simulink model "TRN_V3_2_CodeGen"  (R2022a)
settings: Solver=FixedStepAuto  StartTime=0.0  StopTime=300  FixedStep=0.04  RelTol=1e-3
PreLoadFcn:
  | load('BusStructureTRNsensor.mat');
  | addpath('C:/MAP');
InitFcn:
  | %load TRNDataBusPILS.mat
  | %addpath(genpath(cd))
  | 
  | %load('TPF_WHOLESIM_INPUT_SCENARIOS_AGCAS_N35_10E127_70.mat');
  | 
  | % Add DataBus Path
  | addpath(',,/');
  | addpath('../MAP/');
  | addpath('../MAP/MAP_DB');
  | addpath('../MAP/DVOF');
  | addpath(genpath(cd));
  | load('BusStructureTRN.mat');
undefined symbols (not defined in the file or in its folder): Altitude_INS, Latitude_INS, Longitude_INS, TRN, TRNlib
libraries: simulink_extras x23, aerolibconvert2 x6, sharedtransform x4, dspstat3 x2
(part 2 of 3)

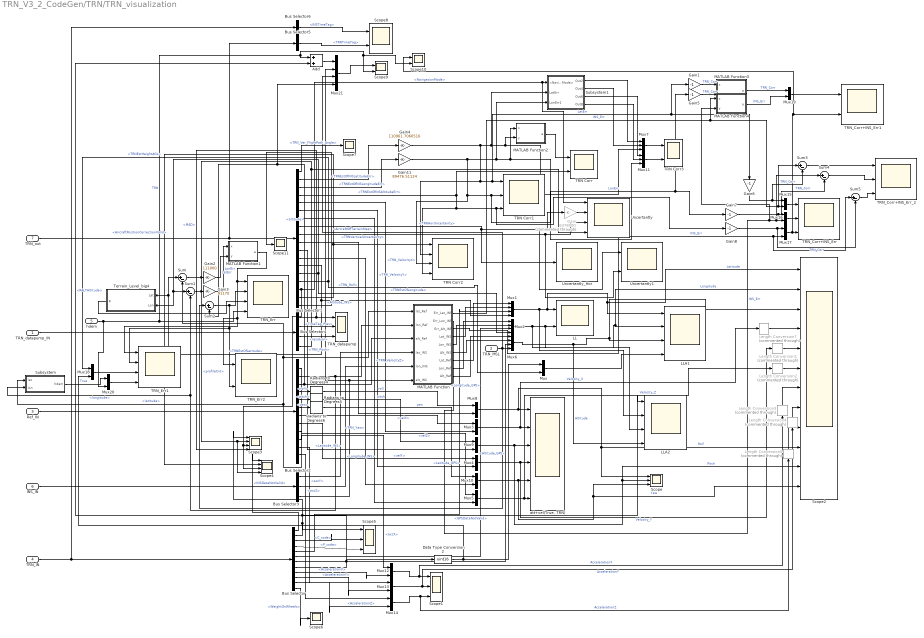
== system TRN_V3_2_CodeGen/TRN/TRN_visualization  ==
  TRN_datapump_IN : Inport
  TRN_MSL : Inport  Port=2
  Ref_IN : Inport  Port=3
  TRN_IN : Inport  Port=4
  hdem : Inport  Port=5
  INS_IN : Inport  Port=6
  TRN_out : Inport  Port=7
  Add : Sum
  Bus Selector : BusSelector  OutputSignals=INSDataNotValid,GPSDataNotValid,C_code,P_code,Latitude_GPS,Longitude_GPS,Altitude_GPS,RALTAltitude,AccelerationX,AccelerationY,AccelerationZ,WeightOnWheels
  Bus Selector1 : BusSelector  OutputSignals=TRN_Ver_FlightPath_Angle,TRNEstOfINSLatitudeErr,TRNEstOfINSLongitudeErr,TRNEstOfINSAltitudeErr,TRN_VelocityX,TRN_VelocityY,TRN_VelocityZ,TRNHorUncertainty,TRNVerticalUncertainty,TRN_Roll,TRN_Pitch,TRN_Yaw,TRNEstOfLatitude,TRNEstOfLongitude,TRNEstHeightAGL,NavigationMode,AircraftPositionCorrectionValid,AircraftOffTerrainMap
  Bus Selector2 : BusSelector  OutputSignals=latitude,longitude,altitude,roll,pitch,yaw,velX,velY,velZ,accX,accY,accZ
  Bus Selector3 : BusSelector  OutputSignals=Latitude_INS,Longitude_INS,Altitude_INS
  Bus Selector4 : BusSelector  OutputSignals=MAD,TimeTag_Prev,residual,profileCnt
  Bus Selector5 : BusSelector  OutputSignals=TRNTimeTag
  Bus Selector6 : BusSelector  OutputSignals=INSTimeTag
  Data Type Conversion2 : DataTypeConversion  OutDataTypeStr=uint16  SaturateOnIntegerOverflow=off  RndMeth=Floor
  Gain : Gain  Commented=through  Gain=6378000
  Gain{1,5..8} (5 alike) : Gain  Gain=-1
  Gain11 : Gain  Gain=89476.51124
  Gain2 : Gain  Gain=111000
  Gain3 : Gain  Gain=91170
  Gain4 : Gain  Gain=110961.7060516
  LL : Scope  NumInputPorts=2
  LLA1 : Scope  NumInputPorts=4
  LLA2 : Scope  NumInputPorts=4
  Length Conversion{1..5,7} (6 alike) : aerolibconvert2/Length Conversion  Commented=through  IU=m  OU=ft
  MATLAB Function : MATLAB Function  TreatAsAtomicUnit=on
  MATLAB Function1 : MATLAB Function  TreatAsAtomicUnit=on
  MATLAB Function2 : MATLAB Function  TreatAsAtomicUnit=on
  MATLAB Function3 : MATLAB Function  TreatAsAtomicUnit=on
  MATLAB Function4 : MATLAB Function  TreatAsAtomicUnit=on
  Mux{,3..5,8..10,12..20} (16 alike) : Mux  Inputs=2
  Mux{1..2,6,21} (4 alike) : Mux
  Mux11 : Mux  Inputs=3
  Mux7 : Mux  Inputs=3
  Radians to Degrees4 : simulink_extras/Transformations/Radians to Degrees
  Radians to Degrees5 : simulink_extras/Transformations/Radians to Degrees
  Radians to Degrees6 : simulink_extras/Transformations/Radians to Degrees
  Scope : Scope  NumInputPorts=3
  Scope1 : Scope  NumInputPorts=3
  Scope10 : Scope  NumInputPorts=2
  Scope11 : Scope
  Scope2 : Scope  NumInputPorts=12
  Scope3 : Scope  NumInputPorts=4
  Scope4 : Scope  NumInputPorts=4
  Scope5 : Scope  NumInputPorts=3
  Scope6 : Scope
  Scope7 : Scope
  Scope8 : Scope  NumInputPorts=2
  Scope9 : Scope  NumInputPorts=2
  Subsystem : Subsystem
  Subsystem1 : Subsystem
  Sum{,1..5} (6 alike) : Sum  Inputs=|+-
  TRN Corr : Scope  NumInputPorts=2
  TRN Corr1 : Scope  NumInputPorts=3
  TRN Corr2 : Scope  NumInputPorts=4
  TRN Corr3 : Scope  NumInputPorts=2
  TRN_Corr+INS_Err : Scope  NumInputPorts=3
  TRN_Corr+INS_Err1 : Scope  NumInputPorts=2
  TRN_Corr+INS_Err_2 : Scope  NumInputPorts=3
  TRN_Err : Scope  NumInputPorts=4
  TRN_Err1 : Scope  NumInputPorts=4
  TRN_Err2 : Scope  NumInputPorts=2
  TRN_datapump : Scope  NumInputPorts=3
  Terrain_Level_big4 : MATLAB Function  TreatAsAtomicUnit=on
  Uncertantly : Scope  NumInputPorts=4
  Uncertantly1 : Scope  NumInputPorts=2
  Uncertantly_Hor : Scope
  "att+vel(True, TRN)" : Scope  NumInputPorts=6
  wires:
  Sum3/1 -> TRN_Corr+INS_Err_2/1
  Sum4/1 -> TRN_Corr+INS_Err_2/2
  Sum5/1 -> TRN_Corr+INS_Err_2/3
  Gain8/1 -> Mux17/1, Sum5/2  "TRN_Corr"
  Gain7/1 -> Mux16/1, Sum4/2  "TRN_Corr"
  Gain6/1 -> Mux15/1, Sum3/2  "TRN_Corr"
  MATLAB Function/3(Err_Alt_INS) -> Mux17/2, Sum5/1  "INS_Err"
  Mux17/1 -> Scope10/1, TRN_Corr+INS_Err1/2, TRN_Corr+INS_Err/3
  MATLAB Function/2(Err_Lon_INS) -> Mux16/2, Sum4/1, MATLAB Function4/2(y)  "INS_Err"
  Mux16/1 -> TRN_Corr+INS_Err/2
  Mux15/1 -> TRN_Corr+INS_Err/1
  MATLAB Function/1(Err_Lat_INS) -> Mux15/2, Sum3/1, MATLAB Function4/1(x)  "INS_Err"
  Bus Selector/4 -> Scope5/3  "<P_code>"
  Bus Selector/3 -> Scope5/2  "<C_code>"
  Bus Selector/7 -> Mux6/3  "<Altitude_GPS>"
  Bus Selector/6 -> Mux2/3  "<Longitude_GPS>"
  Bus Selector/5 -> Mux1/3  "<Latitude_GPS>"
  Length Conversion5/1 -> Scope2/9
  Length Conversion4/1 -> Scope2/8
  Length Conversion3/1 -> Scope2/7
  Length Conversion2/1 -> Scope2/6
  Length Conversion1/1 -> Scope2/5
  Length Conversion7/1 -> Scope2/4
  Bus Selector/1 -> Scope4/1  "<INSDataNotValid>"
  Bus Selector4/4 -> Uncertantly/4, Scope3/2, Scope4/4  "<profileCnt>"
  MATLAB Function1/1(a) -> TRN_Err2/1, TRN_Err1/1, TRN_Err/1
  Bus Selector/2 -> Scope3/1, LLA2/1, Scope5/1  "<GPSDataNotValid>"
  hdem/1 -> Mux20/2, Scope10/2, Scope9/2, Add/1, TRN_Err/4  "TRN"
  Terrain_Level_big4/1(R) -> TRN_Err/3
  Bus Selector1/17 -> TRN Corr2/1, Scope4/2  "<AircraftPositionCorrectionValid>"
  Bus Selector1/5 -> Mux3/2  "<TRN_VelocityX>"
  Mux14/1 -> Scope1/3, Length Conversion5/1  "AccelerationZ"
  Bus Selector/11 -> Mux14/2  "<AccelerationZ>"
  Bus Selector2/12 -> Mux14/1  "<accZ>"
  Bus Selector2/11 -> Mux13/1  "<accY>"
  Bus Selector/10 -> Mux13/2  "<AccelerationY>"
  Mux13/1 -> Scope1/2, Length Conversion4/1  "AccelerationY"
  Bus Selector/9 -> Mux12/2  "<AccelerationX>"
  Bus Selector2/10 -> Mux12/1  "<accX>"
  Mux12/1 -> Scope1/1, Length Conversion3/1  "AccelerationX"
  Mux6/1 -> LLA1/3, Scope2/3, LLA2/4  "Altitude"
  Mux/1 -> LLA1/4
  TRN_IN/1 -> Bus Selector/1, Bus Selector6/1
  Ref_IN/1 -> Bus Selector2/1
  TRN_out/1 -> Bus Selector5/1, Bus Selector1/1
  Gain3/1 -> MATLAB Function1/1(x)  "LonErr"
  Subsystem1/1(Out2) -> Mux7/1
  Mux11/1 -> TRN Corr3/2
  Bus Selector1/9 -> Uncertantly/3, Uncertantly1/2  "<TRNVerticalUncertainty>"
  Bus Selector1/14 -> Mux2/4, Sum1/1, Terrain_Level_big4/2(Lon)  "<TRNEstOfLongitude>"
  Radians to Degrees5/1 -> Mux9/1  "pitch"
  Radians to Degrees4/1 -> Mux8/1  "roll"
  Bus Selector2/7 -> Mux3/1  "<velX>"
  MATLAB Function/6(Alt_INS) -> Mux6/2
  Bus Selector1/12 -> Mux10/2  "<TRN_Yaw>"
  Bus Selector1/11 -> Mux9/2  "<TRN_Pitch>"
  Mux3/1 -> "att+vel(True, TRN)"/2, Length Conversion7/1  "Velocity_X"
  Bus Selector1/10 -> Mux8/2  "<TRN_Roll>"
  Bus Selector3/3 -> Mux21/2, MATLAB Function/6(alt_INS)  "<Altitude_INS>"
  Bus Selector2/9 -> Mux5/1  "<velZ>"
  Mux4/1 -> "att+vel(True, TRN)"/4, Length Conversion1/1  "Velocity_Y"
  Mux1/1 -> LL/1, LLA1/1, Scope2/1, LLA2/2  "Latitude"
  Mux5/1 -> "att+vel(True, TRN)"/6, Length Conversion2/1  "Velocity_Z"
  Bus Selector2/3 -> MATLAB Function/3(alt_Ref), Mux21/4, Sum2/2  "<altitude>"
  Bus Selector1/4 -> TRN Corr2/4, TRN Corr1/3, Gain8/1, TRN Corr/2  "<TRNEstOfINSAltitudeErr>"
  TRN_datapump_IN/1 -> Bus Selector4/1
  Mux2/1 -> LL/2, LLA1/2, Scope2/2, LLA2/3  "Longitude"
  MATLAB Function/9(Alt_Ref) -> Mux6/1
  Gain11/1 -> Mux11/3, MATLAB Function2/1(x), Subsystem1/3(LonErr1), TRN Corr1/2, Gain7/1, Gain5/1, TRN Corr2/3  "LonErr"
  MATLAB Function/4(Lat_INS) -> Mux1/2
  Bus Selector3/2 -> MATLAB Function/5(lon_INS)  "<Longitude_INS>"
  Radians to Degrees6/1 -> Mux10/1  "yaw"
  Bus Selector4/2 -> TRN_datapump/2  "<TimeTag_Prev>"
  MATLAB Function/8(Lon_Ref) -> Mux2/1
  Bus Selector2/6 -> Radians to Degrees6/1  "<yaw>"
  MATLAB Function2/1(a) -> TRN Corr/1
  Bus Selector/8 -> Add/2, Data Type Conversion2/1  "<RALTAltitude>"
  Bus Selector1/16 -> Scope3/3, Scope4/3, Uncertantly/1, Subsystem1/1(<NavigationMode>)  "<NavigationMode>"
  Sum2/1 -> TRN_Err1/2, TRN_Err2/2, TRN_Err/2
  Bus Selector2/5 -> Radians to Degrees5/1  "<pitch>"
  Mux7/1 -> TRN Corr3/1
  INS_IN/1 -> Bus Selector3/1
  Bus Selector4/1 -> TRN_datapump/1, Scope3/4  "<MAD>"
  Bus Selector1/3 -> Gain11/1  "<TRNEstOfINSLongitudeErr>"
  Bus Selector1/6 -> Mux4/2  "<TRN_VelocityY>"
  Bus Selector3/1 -> MATLAB Function/4(lat_INS)  "<Latitude_INS>"
  Subsystem1/3(Out6) -> Mux11/1
  Mux8/1 -> "att+vel(True, TRN)"/1, Scope/1, Scope2/10  "Roll"
  TRN_MSL/1 -> Mux21/3, Sum2/1, Mux6/4
  Bus Selector1/15 -> Mux/2, Mux18/1  "<TRNEstHeightAGL>"
  MATLAB Function/7(Lat_Ref) -> Mux1/1
  Mux9/1 -> "att+vel(True, TRN)"/3, Scope/2, Scope2/11  "Pitch"
  Subsystem1/2(Out4) -> Mux7/2
  Sum1/1 -> Gain3/1
  Bus Selector1/7 -> Mux5/2  "<TRN_VelocityZ>"
  Bus Selector1/2 -> Gain4/1  "<TRNEstOfINSLatitudeErr>"
  Bus Selector2/2 -> Subsystem/2(lon), Sum1/2, MATLAB Function/2(lon_Ref)  "<longitude>"
  Subsystem1/4(Out8) -> Mux11/2
  Gain2/1 -> MATLAB Function1/2(y)  "LatErr"
  Gain4/1 -> Mux7/3, MATLAB Function2/2(y), Subsystem1/2(LatErr), TRN Corr1/1, Gain6/1, Gain1/1, TRN Corr2/2  "LatErr"
  Bus Selector2/8 -> Mux4/1  "<velY>"
  MATLAB Function/5(Lon_INS) -> Mux2/2
  Bus Selector4/3 -> TRN_datapump/3  "<residual>"
  Bus Selector1/8 -> Uncertantly_Hor/1, Gain/1, Uncertantly1/1  "<TRNHorUncertainty>"
  Sum/1 -> Gain2/1
  Mux10/1 -> "att+vel(True, TRN)"/5, Scope2/12, Scope/3  "Yaw"
  Bus Selector2/1 -> MATLAB Function/1(lat_Ref), Sum/2, Subsystem/1(lat)  "<latitude>"
  Bus Selector2/4 -> Radians to Degrees4/1  "<roll>"
  Bus Selector1/13 -> Sum/1, Terrain_Level_big4/1(Lat), Mux1/4  "<TRNEstOfLatitude>"
  Bus Selector/12 -> Scope6/1  "<WeightOnWheels>"
  Bus Selector1/1 -> Scope7/1  "<TRN_Ver_FlightPath_Angle>"
  Mux18/1 -> TRN_Err1/3
  Data Type Conversion2/1 -> Mux/1, Mux18/2
  Mux19/1 -> TRN_Corr+INS_Err1/1
  MATLAB Function4/1(a) -> Mux19/2  "INS_Err"
  MATLAB Function3/1(a) -> Mux19/1  "TRN_Corr"
  Gain1/1 -> MATLAB Function3/1(x)  "TRN_Corr"
  Gain5/1 -> MATLAB Function3/2(y)  "TRN_Corr"
  Mux20/1 -> TRN_Err1/4
  Subsystem/1(hdem) -> Mux20/1  "True"
  Bus Selector6/1 -> Scope8/1  "<INSTimeTag>"
  Bus Selector5/1 -> Scope8/2  "<TRNTimeTag>"
  Add/1 -> Mux21/1
  Mux21/1 -> Scope9/1
  Gain/1 -> Uncertantly/2
  Bus Selector1/18 -> Scope11/1  "<AircraftOffTerrainMap>"

== system TRN_V3_2_CodeGen/TRN/Terrain_Func ==
  lat : Inport
  lon : Inport  Port=2
  CheckOffTerrainMap : MATLAB Function  TreatAsAtomicUnit=on
  MATLAB Function : MATLAB Function  Commented=on  TreatAsAtomicUnit=on
  Terminator : Terminator
  Terrain_roughness : MATLAB Function  TreatAsAtomicUnit=on
  UpdateCache : MATLAB Function  TreatAsAtomicUnit=on
  updateFlag : MATLAB Function  TreatAsAtomicUnit=on
  hdem : Outport
  Updateflag : Outport  Port=2
  AircraftOffTerrainMap : Outport  Port=3
  wires:
  lat/1 -> UpdateCache/1(lat), Terrain_roughness/1(Lat)
  UpdateCache/2(hDEM) -> CheckOffTerrainMap/1(hDEM), hdem/1
  lon/1 -> UpdateCache/2(lon), Terrain_roughness/2(Lon)
  Terrain_roughness/1(R) -> updateFlag/2(roughness)
  updateFlag/1(UpdateFlag) -> Updateflag/1
  CheckOffTerrainMap/1(AircraftOffTerrainMap) -> updateFlag/1(AircraftOffTerrainMap), AircraftOffTerrainMap/1
  UpdateCache/1(result) -> Terminator/1

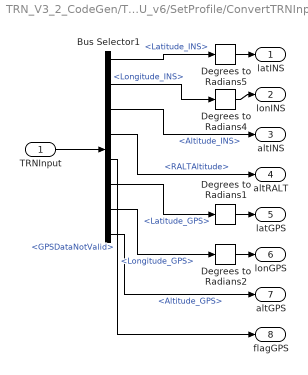
== system TRN_V3_2_CodeGen/TRN/ModeManagementCSU_v6/SetProfile/ConvertTRNInput ==
  TRNInput : Inport  OutDataTypeStr=Bus: TRNInput
  Bus Selector1 : BusSelector  OutputSignals=Latitude_INS,Longitude_INS,Altitude_INS,RALTAltitude,GPSDataNotValid,Latitude_GPS,Longitude_GPS,Altitude_GPS
  Degrees to Radians{1..2,4..5} (4 alike) : simulink_extras/Transformations/Degrees to Radians
  latINS : Outport  VectorParamsAs1DForOutWhenUnconnected=off
  lonINS : Outport  Port=2  VectorParamsAs1DForOutWhenUnconnected=off
  altINS : Outport  Port=3  VectorParamsAs1DForOutWhenUnconnected=off
  altRALT : Outport  Port=4  VectorParamsAs1DForOutWhenUnconnected=off
  latGPS : Outport  Port=5  VectorParamsAs1DForOutWhenUnconnected=off
  lonGPS : Outport  Port=6  VectorParamsAs1DForOutWhenUnconnected=off
  altGPS : Outport  Port=7  VectorParamsAs1DForOutWhenUnconnected=off
  flagGPS : Outport  Port=8  VectorParamsAs1DForOutWhenUnconnected=off
  wires:
  Bus Selector1/2 -> Degrees to Radians4/1  "<Longitude_INS>"
  Bus Selector1/1 -> Degrees to Radians5/1  "<Latitude_INS>"
  Bus Selector1/4 -> altRALT/1  "<RALTAltitude>"
  Degrees to Radians4/1 -> lonINS/1
  Degrees to Radians5/1 -> latINS/1
  TRNInput/1 -> Bus Selector1/1
  Bus Selector1/3 -> altINS/1  "<Altitude_INS>"
  Bus Selector1/5 -> flagGPS/1  "<GPSDataNotValid>"
  Bus Selector1/6 -> Degrees to Radians1/1  "<Latitude_GPS>"
  Bus Selector1/7 -> Degrees to Radians2/1  "<Longitude_GPS>"
  Bus Selector1/8 -> altGPS/1  "<Altitude_GPS>"
  Degrees to Radians2/1 -> lonGPS/1
  Degrees to Radians1/1 -> latGPS/1

== system TRN_V3_2_CodeGen/TRN/ModeManagementCSU_v6/TrackingCSUMeasurement/residualValidCheck2 ==
  TRNDatapump : Inport
  Bus Selector7 : BusSelector  OutputSignals=residual
  Data Type Conversion2 : DataTypeConversion  OutDataTypeStr=boolean  SaturateOnIntegerOverflow=off  RndMeth=Floor
  Gain2 : Gain  Gain=3
  StdDev : MATLAB Function  TreatAsAtomicUnit=on
  Unit Delay3 : UnitDelay  SampleTime=-1  HasFrameUpgradeWarning=on
  residualCheck : MATLAB Function  TreatAsAtomicUnit=on
  residualValid : Outport
  wires:
  Data Type Conversion2/1 -> residualValid/1
  residualCheck/1(residualValid) -> Data Type Conversion2/1
  StdDev/1(std) -> Gain2/1
  Gain2/1 -> residualCheck/2(sigma_3)
  residualCheck/2(count) -> Unit Delay3/1
  TRNDatapump/1 -> Bus Selector7/1
  Unit Delay3/1 -> residualCheck/3("count ")
  Bus Selector7/1 -> StdDev/1(x), residualCheck/1(residual)  "<residual>"

== system TRN_V3_2_CodeGen/TRN/TRN_visualization /Subsystem ==
  lat : Inport
  lon : Inport  Port=2
  MATLAB Function : MATLAB Function  Commented=on  TreatAsAtomicUnit=on
  UpdateCache : MATLAB Function  TreatAsAtomicUnit=on
  hdem : Outport
  wires:
  lat/1 -> UpdateCache/1(lat)
  UpdateCache/2(hDEM) -> hdem/1
  lon/1 -> UpdateCache/2(lon)

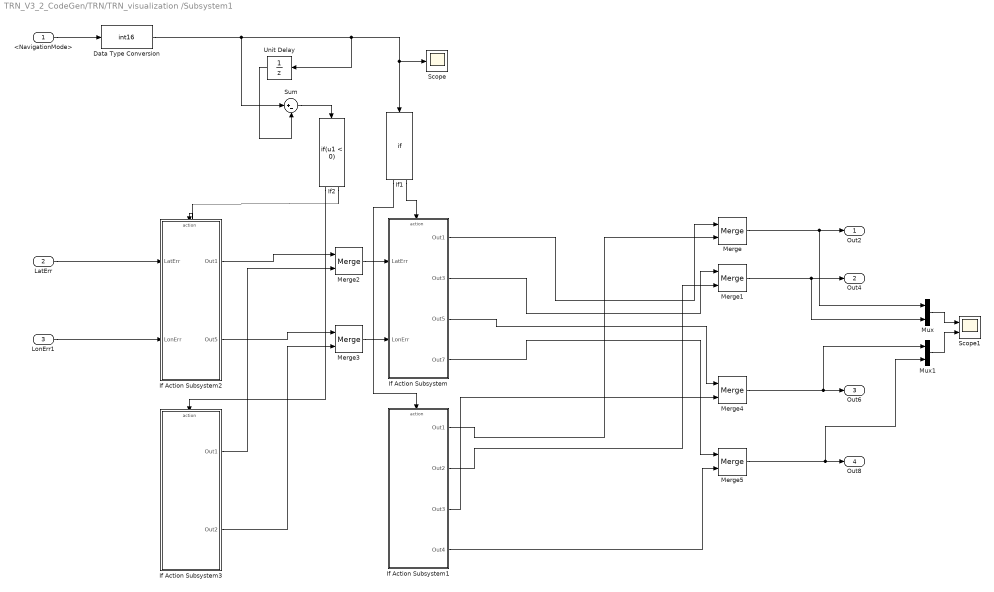
== system TRN_V3_2_CodeGen/TRN/TRN_visualization /Subsystem1 ==
  <NavigationMode> : Inport
  LatErr : Inport  Port=2
  LonErr1 : Inport  Port=3
  Data Type Conversion : DataTypeConversion  OutDataTypeStr=int16  SaturateOnIntegerOverflow=off  RndMeth=Floor
  If Action Subsystem : Subsystem  TreatAsAtomicUnit=on
  If Action Subsystem1 : Subsystem  TreatAsAtomicUnit=on
  If Action Subsystem2 : Subsystem  TreatAsAtomicUnit=on
  If Action Subsystem3 : Subsystem  TreatAsAtomicUnit=on
  If1 : If
  If2 : If  IfExpression=u1 < 0
  Merge{,1..5} (6 alike) : Merge
  Mux : Mux  Inputs=2
  Mux1 : Mux  Inputs=2
  Scope : Scope
  Scope1 : Scope  NumInputPorts=2
  Sum : Sum  Inputs=|+-
  Unit Delay : UnitDelay  SampleTime=-1  HasFrameUpgradeWarning=on
  Out2 : Outport
  Out4 : Outport  Port=2
  Out6 : Outport  Port=3
  Out8 : Outport  Port=4
  wires:
  If Action Subsystem3/2(Out2) -> Merge3/2
  If Action Subsystem2/2(Out5) -> Merge3/1
  If Action Subsystem3/1(Out1) -> Merge2/2
  If Action Subsystem2/1(Out1) -> Merge2/1
  Merge3/1 -> If Action Subsystem/2(LonErr)
  Merge2/1 -> If Action Subsystem/1(LatErr)
  LonErr1/1 -> If Action Subsystem2/2(LonErr)
  LatErr/1 -> If Action Subsystem2/1(LatErr)
  If2/1 -> If Action Subsystem3/Action
  If2/2 -> If Action Subsystem2/Action
  Sum/1 -> If2/1
  Unit Delay/1 -> Sum/2
  Mux1/1 -> Scope1/2
  Mux/1 -> Scope1/1
  <NavigationMode>/1 -> Data Type Conversion/1
  If Action Subsystem1/4(Out4) -> Merge5/2
  If Action Subsystem1/3(Out3) -> Merge4/2
  If Action Subsystem/4(Out7) -> Merge5/1
  If Action Subsystem/3(Out5) -> Merge4/1
  If Action Subsystem/2(Out3) -> Merge1/1
  Merge1/1 -> Out4/1, Mux/2
  Merge/1 -> Out2/1, Mux/1
  If1/1 -> If Action Subsystem1/Action
  If Action Subsystem1/1(Out1) -> Merge/2
  If Action Subsystem1/2(Out2) -> Merge1/2
  Data Type Conversion/1 -> Sum/1, Scope/1, If1/1, Unit Delay/1
  Merge4/1 -> Out6/1, Mux1/1
  Merge5/1 -> Out8/1, Mux1/2
  If1/2 -> If Action Subsystem/Action
  If Action Subsystem/1(Out1) -> Merge/1

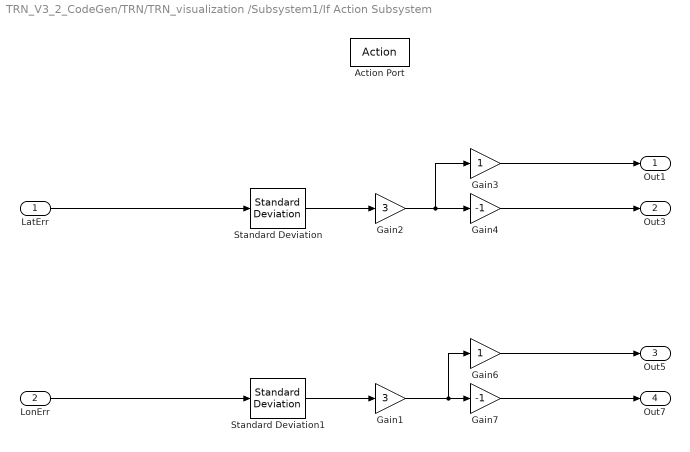
== system TRN_V3_2_CodeGen/TRN/TRN_visualization /Subsystem1/If Action Subsystem ==
  LatErr : Inport
  LonErr : Inport  Port=2
  Action Port : ActionPort
  Gain1 : Gain  Gain=3
  Gain2 : Gain  Gain=3
  Gain3 : Gain
  Gain4 : Gain  Gain=-1
  Gain6 : Gain
  Gain7 : Gain  Gain=-1
  Standard Deviation : dspstat3/Standard Deviation  run=on  directionMode=Entire input  dimension=1  reset_popup=None  roiEnable=off  roiType=Rectangles  roiPortion=Entire ROI  roiOutput=Individual statistics for each ROI  roiFlag=off
      settings: SourceProductBaseCode=DS
  Standard Deviation1 : dspstat3/Standard Deviation  run=on  directionMode=Entire input  dimension=1  reset_popup=None  roiEnable=off  roiType=Rectangles  roiPortion=Entire ROI  roiOutput=Individual statistics for each ROI  roiFlag=off
      settings: SourceProductBaseCode=DS
  Out1 : Outport
  Out3 : Outport  Port=2
  Out5 : Outport  Port=3
  Out7 : Outport  Port=4
  wires:
  LatErr/1 -> Standard Deviation/1
  LonErr/1 -> Standard Deviation1/1
  Gain6/1 -> Out5/1
  Gain2/1 -> Gain4/1, Gain3/1
  Gain7/1 -> Out7/1
  Standard Deviation1/1 -> Gain1/1
  Standard Deviation/1 -> Gain2/1
  Gain3/1 -> Out1/1
  Gain4/1 -> Out3/1
  Gain1/1 -> Gain7/1, Gain6/1

== system TRN_V3_2_CodeGen/TRN/TRN_visualization /Subsystem1/If Action Subsystem1 ==
  Action Port : ActionPort
  Constant : Constant  Value=0
  Out1 : Outport
  Out2 : Outport  Port=2
  Out3 : Outport  Port=3
  Out4 : Outport  Port=4
  wires:
  Constant/1 -> Out4/1, Out3/1, Out2/1, Out1/1

== system TRN_V3_2_CodeGen/TRN/TRN_visualization /Subsystem1/If Action Subsystem2 ==
  LatErr : Inport
  LonErr : Inport  Port=2
  Action Port : ActionPort
  Out1 : Outport
  Out5 : Outport  Port=2
  wires:
  LonErr/1 -> Out5/1
  LatErr/1 -> Out1/1

== system TRN_V3_2_CodeGen/TRN/TRN_visualization /Subsystem1/If Action Subsystem3 ==
  Action Port : ActionPort
  Constant : Constant  Value=0
  Out1 : Outport
  Out2 : Outport  Port=2
  wires:
  Constant/1 -> Out2/1, Out1/1

== matlab function TRN_V3_2_CodeGen/TRN/Terrain_Func/CheckOffTerrainMap ==
  data: hDEM input; AircraftOffTerrainMap output
function AircraftOffTerrainMap = CheckOffTerrainMap(hDEM)

if(hDEM == -1)
    AircraftOffTerrainMap = true;
else
    AircraftOffTerrainMap = false;
end

end

== matlab function TRN_V3_2_CodeGen/TRN/ModeManagementCSU_v6/StoreProfile/SetProfile function ==
  data: batchProfile input; batchProfile output; profileCnt input; profileCnt output; gridSize input; flagINS input
function [batchProfile, profileCnt] = SetProfile(batchProfile, profileCnt, gridSize, flagINS)

if(profileCnt >= 20)
      
    profileCnt = uint32(19);
    
    for i = 0:profileCnt-1
   
        for j = 1 : (3 + (gridSize + gridSize + 1) * (gridSize + gridSize + 1))
            batchProfile(i * (3 + (gridSize + gridSize + 1) * (gridSize + gridSize + 1)) + j) = batchProfile((i+1) * (3 + (gridSize + gridSize + 1) * (gridSize + gridSize + 1)) + j);
        end
    end
            
end

if flagINS == 0
    profileCnt = profileCnt + 1;
else
    profileCnt = uint32(0);
end


end

== matlab function TRN_V3_2_CodeGen/TRN/TRNCorrCheck ==
  data: latINS input; TRNEstOfLatErr output; lonINS input; altINS input; TRNEstOfLonErr output; TRNEstOfaltErr output; roll input; pitch input; GPSDataNotvalid input; NotCorrFlag input; NotCorrFlag output
function [TRNEstOfLatErr, TRNEstOfLonErr, TRNEstOfaltErr,NotCorrFlag] = TRNCorrCheck(latINS, lonINS, altINS, roll, pitch, GPSDataNotvalid, NotCorrFlag)

if GPSDataNotvalid == true
    if abs(roll) > 15 || abs(pitch) > 15
        TRNEstOfLatErr_temp = latINS;
        TRNEstOfLonErr_temp = lonINS;
        TRNEstOfaltErr_temp = altINS;
        TRNEstOfLatErr = TRNEstOfLatErr_temp;
        TRNEstOfLonErr = TRNEstOfLonErr_temp;
        TRNEstOfaltErr = TRNEstOfaltErr_temp;
        NotCorrFlag = 1;
    else
        TRNEstOfLatErr = latINS;
        TRNEstOfLonErr = lonINS;
        TRNEstOfaltErr = altINS;
        TRNEstOfLatErr_temp = 0;
        TRNEstOfLonErr_temp = 0;
        TRNEstOfaltErr_temp = 0;
        NotCorrFlag = 0;
    end
    
    if NotCorrFlag == 1
        TRNEstOfLatErr = TRNEstOfLatErr_temp;
        TRNEstOfLonErr = TRNEstOfLonErr_temp;
        TRNEstOfaltErr = TRNEstOfaltErr_temp;
    end
else
    TRNEstOfLatErr = latINS;
    TRNEstOfLonErr = lonINS;
    TRNEstOfaltErr = altINS;
    NotCorrFlag = 0;
end

== matlab function TRN_V3_2_CodeGen/TRN/TRNvalidCheck ==
  data: INS_Mech_flag input; TRN_valid output; Latitude_INS input
function TRN_valid = TRNvalidCheck(INS_Mech_flag, Latitude_INS)

    if( abs(Latitude_INS) > 80.0)
        Latitude_INS_flag = 0;
    else
        Latitude_INS_flag = 1;
    end

    if( (INS_Mech_flag < 1) || (Latitude_INS_flag < 1))
        TRN_valid = boolean(false);
    else
        TRN_valid = boolean(true);
    end

end

== matlab function TRN_V3_2_CodeGen/TRN/Terrain_Func/MATLAB Function ==
  data: Resolution output; Map_Size output; bottomLat output; leftLon output
function [Resolution, Map_Size, bottomLat, leftLon] = ReturnBottomLeftLatLon

Resolution = double(0.0);
Map_Size = double(0.0);

leftLon = 0.0;
leftLon = coder.ceval('ReturnLeftLon');

bottomLat = 0.0;
bottomLat = coder.ceval('ReturnBottomLat');

end

== matlab function TRN_V3_2_CodeGen/TRN/TRN_visualization /MATLAB Function ==
  data: Err_Lat_INS output; Err_Lon_INS output; Err_Alt_INS output; lat_Ref input; lon_Ref input; alt_Ref input; lat_INS input; lon_INS input; alt_INS input; Lat_INS output; Lon_INS output; Alt_INS output; Lat_Ref output; Lon_Ref output; Alt_Ref output
function [Err_Lat_INS, Err_Lon_INS, Err_Alt_INS, Lat_INS, Lon_INS, Alt_INS, Lat_Ref, Lon_Ref, Alt_Ref] = fcn(lat_Ref, lon_Ref, alt_Ref, lat_INS, lon_INS, alt_INS)

%% parameters
lat2m = 110961.7060516;
lon2m = 89476.51124;

%% 초기값 setting
% init_lat = 35.1;
% init_lon = 128.5;
% init_alt = 1000;

Lat_INS = lat_INS;               % INS Latitude
Lon_INS = lon_INS;               % INS Longitude
% Alt_INS = uint16(alt_INS);               % INS Altitude
Alt_INS = alt_INS;               % INS Altitude

Lat_Ref = lat_Ref;             % Ref Latitude
Lon_Ref = lon_Ref;             % Ref Longitude
% Alt_Ref = uint16(alt_Ref);             % Ref Altitude
Alt_Ref = alt_Ref;             % Ref Altitude

Err_Lat_INS = (Lat_Ref-Lat_INS)*lat2m;
Err_Lon_INS = (Lon_Ref-Lon_INS)*lon2m;
Err_Alt_INS = (Alt_Ref-Alt_INS);

end

== matlab function TRN_V3_2_CodeGen/TRN/TRN_visualization /MATLAB Function1 ==
  data: x input; a output; y input
function a = fcn(x,y)

a = sqrt(x^2+y^2);

== matlab function TRN_V3_2_CodeGen/TRN/TRN_visualization /MATLAB Function2 ==
  data: x input; a output; y input
function a = fcn(x,y)

a = sqrt(x^2+y^2);

== matlab function TRN_V3_2_CodeGen/TRN/TRN_visualization /Terrain_Level_big4 ==
  data: Lat input; Lon input; R output
function R = Terrain_level_big1(Lat, Lon)

    R = Terrain_level(Lat, Lon);

end

== matlab function TRN_V3_2_CodeGen/TRN/GPSmode_Uncertainty_init/Uncertainty_init ==
  data: P input; hUncertainty output; vUncertainty output
function [hUncertainty,vUncertainty] = Uncertainty_init(P)

hUncertainty = sqrt(abs(P(7,7) + P(8,8))) * 6378000;
vUncertainty = sqrt(abs(P(9,9)));

== matlab function TRN_V3_2_CodeGen/TRN/ModeManagementCSU_v6/CorrelationValid/CorrelationValid function ==
  data: posUpdate input; MAD input; profileCnt input; TRNEstOfINSLatitudeErr output; TRNEstOfINSLongitudeErr output; TRNEstOfINSAltitudeErr output; GPSDataNotValid input; profileCnt output; NavigationMode output; AircraftPositionCorrectionValid output
function [TRNEstOfINSLatitudeErr, TRNEstOfINSLongitudeErr, TRNEstOfINSAltitudeErr, profileCnt, NavigationMode, AircraftPositionCorrectionValid] = CorrelationValid(posUpdate, MAD, profileCnt, GPSDataNotValid)

if (MAD < 50 && profileCnt >= 20) || ...
 (GPSDataNotValid == 0 && MAD < 50 && profileCnt >= 5)
    TRNEstOfINSLatitudeErr = -posUpdate(1) * 180/pi;
    TRNEstOfINSLongitudeErr = -posUpdate(2) * 180/pi;
    TRNEstOfINSAltitudeErr = 0.0;
    profileCnt = uint32(0);
    NavigationMode = false;
    AircraftPositionCorrectionValid = true;
else
    TRNEstOfINSLatitudeErr = 0.0;
    TRNEstOfINSLongitudeErr = 0.0;
    TRNEstOfINSAltitudeErr = 0.0;
    NavigationMode = true;
    AircraftPositionCorrectionValid = false;
end
end

== matlab function TRN_V3_2_CodeGen/TRN/ModeManagementCSU_v6/SetProfile/SetProfile function ==
  data: batchProfile output; latINS input; lonINS input; altINS input; RALT input; latGPS input; lonGPS input; altGPS input; flagGPS input; profileCnt input; batchProfile input; gridSize input
function batchProfile   = SetProfile(latINS, lonINS, altINS, RALT, latGPS, lonGPS, altGPS, flagGPS, profileCnt, batchProfile, gridSize)

if flagGPS == true
    batchProfile((profileCnt*(3+((gridSize + gridSize + 1) * (gridSize + gridSize + 1)))) + 1) = altINS - RALT;
    batchProfile((profileCnt*(3+((gridSize + gridSize + 1) * (gridSize + gridSize + 1)))) + 2) = latINS;
    batchProfile((profileCnt*(3+((gridSize + gridSize + 1) * (gridSize + gridSize + 1)))) + 3) = lonINS;
else
    batchProfile((profileCnt*(3+((gridSize + gridSize + 1) * (gridSize + gridSize + 1)))) + 1) = altGPS - RALT;
    batchProfile((profileCnt*(3+((gridSize + gridSize + 1) * (gridSize + gridSize + 1)))) + 2) = latGPS;
    batchProfile((profileCnt*(3+((gridSize + gridSize + 1) * (gridSize + gridSize + 1)))) + 3) = lonGPS;
end



end

== matlab function TRN_V3_2_CodeGen/TRN/ModeManagementCSU_v6/TrackingCSUEKFUpdate/EKFUpdate ==
  data: GPSDataNotValid input; zmat_TRN input; zmat_GPS input; xu output; P output; Fmatrix input; Hmat_TRN input; Hmat_GPS input; Gmatrix input; P input; Q input; Rmat_TRN input; Rmat_GPS input; dt input; residual output; latINSErrTRN output; lonINSErrTRN output; altINSErrTRN output; xu_prev input; TimeTag_Prev input; GPSflag input; GPSHorUncert input; GPSVerUncert input; hUncertainty output; vUncertainty output
function [xu, P, residual, latINSErrTRN, lonINSErrTRN, altINSErrTRN, hUncertainty, vUncertainty] ...
    = EKFUpdate(GPSDataNotValid, zmat_TRN, zmat_GPS, Fmatrix, Hmat_TRN, Hmat_GPS, Gmatrix, P, Q, Rmat_TRN, Rmat_GPS, dt, xu_prev, TimeTag_Prev, GPSflag, GPSHorUncert, GPSVerUncert)

x = zeros(15,1);
I = eye(max(size(Fmatrix)));

A = I + (Fmatrix*dt);
Q = (A*Gmatrix * Q * Gmatrix'*A') .* dt;

%-------------------------------------%
% Predicts states & covariance matrix
%-------------------------------------%
xp = A * x;
Pp = (A * P * A') + Q;

%--------------------------------------------------------%
% TRN
if GPSflag > 1 || GPSDataNotValid == true
    K = (Pp * Hmat_TRN')/(Rmat_TRN + Hmat_TRN * Pp * Hmat_TRN');
    xu = xp + K * (zmat_TRN - Hmat_TRN*xp);
    residual = zmat_TRN;
    P = (I - K*Hmat_TRN) * Pp * (I - K*Hmat_TRN)' + K*Rmat_TRN*K';

    hUncertainty = sqrt(abs(P(7,7) + P(8,8))) * 6378000;    % unit m
    vUncertainty = sqrt(abs(P(9,9)));                       % unit m
%--------------------------------------------------------%
% GPS
else
    K = (Pp * Hmat_GPS')/(Rmat_GPS + Hmat_GPS * Pp * Hmat_GPS');
    xu = xp + K * (zmat_GPS - Hmat_GPS*xp);
    residual = zmat_GPS(3);
    P = (I - K*Hmat_GPS) * Pp * (I - K*Hmat_GPS)' + K*Rmat_GPS*K';
    
    hUncertainty = double(GPSHorUncert);     % unit m
    vUncertainty = double(GPSVerUncert);     % unit m
end
%--------------------------------------------------------%

%---------------------------%
% Updates covariance matrix
%---------------------------%
% P = (I - K*H) * Pp * (I - K*H)' + K*R*K';

latINSErrTRN = xu(7);
lonINSErrTRN = xu(8);
altINSErrTRN = xu(9);

%--------------------------------------------------------%
% TRN
if GPSflag > 1 || GPSDataNotValid == true
    if (TimeTag_Prev(6) == 1)
        xu = xu_prev;
        latINSErrTRN = xu(7);
        lonINSErrTRN = xu(8);
        altINSErrTRN = xu(9);
    end
%--------------------------------------------------------%
% GPS
else
    if (TimeTag_Prev(4) == 1)
        xu = xu_prev;
        latINSErrTRN = xu(7);
        lonINSErrTRN = xu(8);
        altINSErrTRN = xu(9);
    end
end
%--------------------------------------------------------%
end

== matlab function TRN_V3_2_CodeGen/TRN/ModeManagementCSU_v6/TrackingCSUTimeTag/INS_Update_1553falt ==
  data: latINS input; latINS output; lonINS input; altINS input; velN input; velE input; velD input; TimeTag input; lonINS output; altINS output; dt input
function [latINS, lonINS, altINS] = INS_Update_1553falt(latINS, lonINS, altINS, velN, velE, velD, TimeTag, dt)

R0 = 6378000;

if TimeTag(5) == 1
    latINS = latINS + (velN * dt) * 1/(R0+altINS);
    lonINS = lonINS + (velE * dt) * 1/(R0+altINS);
    altINS = altINS + (velD * dt) * 1/(R0+altINS);
end

== matlab function TRN_V3_2_CodeGen/TRN/ModeManagementCSU_v6/TrackingCSUTimeTag/TimeTagCheck ==
  data: TimeTag_Prev input; TimeTag_Prev output; GPStimeValid input; INSTimeTag input; RALTTimeTag input
function TimeTag_Prev   = TimeTagCheck(TimeTag_Prev,GPStimeValid,INSTimeTag,RALTTimeTag)


TimeTag_Prev(4) = 0;
TimeTag_Prev(5) = 0;
TimeTag_Prev(6) = 0;

if TimeTag_Prev(1) == GPStimeValid
    TimeTag_Prev(4) = 1;
end

if TimeTag_Prev(2) == INSTimeTag
    TimeTag_Prev(5) = 1;
end

if TimeTag_Prev(3) == RALTTimeTag
    TimeTag_Prev(6) = 1;
end

TimeTag_Prev(1) = GPStimeValid;
TimeTag_Prev(2) = INSTimeTag;
TimeTag_Prev(3) = RALTTimeTag;

== matlab function TRN_V3_2_CodeGen/TRN/ModeManagementCSU_v6/FmatGmatUpdate/Earth_radius ==
  data: M output; N output; Latitude_INS input; psi output
function [M, N, psi] = Earth_radius(Latitude_INS)

    a   = 6378137;          % Earth's equatorial radius
    b   = 6356752.314245;   % Earth's polar radius
    psi = Latitude_INS;     % psi(latitude_INS)
    M   = ((a*b)^2) / ( ( (a*cos(psi))^2 + (b*sin(psi))^2 )^(3/2) );    % radius  of  curvature  in  meridian
    N   = (a^2) / ( ( (a*cos(psi))^2 + (b*sin(psi))^2 )^(1/2) );        % radius  of  curvature  in  prime  vertical

end

== matlab function TRN_V3_2_CodeGen/TRN/ModeManagementCSU_v6/FmatGmatUpdate/Fupdate ==
  data: lat input; alt input; velN input; Fmatrix output; velE input; velD input; accN input; accE input; accD input; OM input; M input; N input; DCMbn input
% ---------------------------------------------------------------------- %
%                   F matrix update function
%
%   INPUT:
%       lat: Latitude                                       [rad]
%       alt: Altitude                                       [m]
%       velN: North Velocity                                [m/s]
%       velE: East Velocity                                 [m/s]
%       velD: Down Velocity                                 [m/s]
%       accN: North acceleration                            [m/ss]
%       accE: East acceleration                             [m/ss]
%       accD: Down acceleration                             [m/ss]
%       OM: Magnitude of the rotation rate of the Earth     [rad/s]
%       R0: Radius of Earth                                 [m]
%       DCMbn: Rotational matrix(body frame to navigation frame)
%
%   OUTPUT:
%       Fmatrix: System matrix of Kalman Filter
%
% ---------------------------------------------------------------------- %
function Fmatrix = Fupdate(lat, alt, velN, velE, velD, accN, accE, accD, OM, M, N, DCMbn)
    
        Z  = zeros(3);
    
        e11 = 0;
        e12 = -((OM * sin(lat)) + (velE/(N+alt) * tan(lat)));
        e13 = velN/(M+alt);
        e21 = ((OM * sin(lat)) + (velE/(N+alt) * tan(lat)));
        e22 = 0;
        e23 = ((OM * cos(lat)) + (velE/(N+alt)));
        e31 = -velN/(M+alt);
        e32 = -(OM * cos(lat)) - (velE/(N+alt));
        e33 = 0;
        Fee = [e11 e12 e13; e21 e22 e23; e31 e32 e33;];
    
        e11 = 0;
        e12 = 1/((N+alt));
        e13 = 0;
        e21 = -1/((M+alt));
        e22 = 0 ;
        e23 = 0 ;
        e31 = 0 ;
        e32 = -tan(lat)/(N+alt) ;
        e33 = 0 ;
        Fev = [e11 e12 e13; e21 e22 e23; e31 e32 e33;];
    
        e11 = -OM * sin(lat);
        e12 = 0;
        e13 = -velE/(((N+alt))^2);
        e21 = 0 ;
        e22 = 0 ;
        e23 = velN/(((M+alt))^2);
        e31 =  -(OM*cos(lat)) - (velE/(((N+alt))*(cos(lat))^2));
        e32 = 0 ;
        e33 = (velE * tan(lat)) / ((N+alt)^2) ;
        Fep = [e11 e12 e13; e21 e22 e23; e31 e32 e33;];
    
        e11 = 0 ;
        e12 = -accD ;
        e13 = accE ;
        e21 = accD ;
        e22 = 0 ;
        e23 = -accN ;
        e31 = -accE ;
        e32 = accN ;
        e33 = 0 ;
        Fve = [e11 e12 e13; e21 e22 e23; e31 e32 e33;];
    
        e11 = velD/((M+alt));
        e12 = -2*((OM * sin(lat)) + ((velE/((N+alt))) * tan (lat))) ;
        e13 = velN/(M+alt) ;
        e21 = (2*OM * sin(lat)) + ( (velE/((N+alt))) * tan(lat) );
        e22 = (1/((N+alt))) * ((velN * tan(lat)) + velD) ;
        e23 = 2*OM * cos(lat) + (velE/((N+alt)));
        e31 = (-2*velN)/((M+alt));
        e32 = -2*(OM * cos(lat) +  (velE/((N+alt)))) ;
        e33 = 0;
        Fvv = [e11 e12 e13; e21 e22 e23; e31 e32 e33;];
    
        e11 = -velE*( (2*OM * cos(lat)) + (velE/(((N+alt))*(cos(lat))^2)));
        e12 = 0 ;
        e13 = (((velE^2)*tan(lat))/((N+alt)^2)) - ((velN*velD)/((M+alt)^2)) ;
        e21 = 2*OM *((velN*cos(lat)) - (velD*sin(lat))) + ((velN*velE) / (((N+alt))*(cos(lat))^2)) ;
        e22 = 0 ;
        e23 = ((-velE*velD)/((N+alt)^2))-((velN*velE*tan(lat))/((N+alt)^2));
        e31 = 2 * OM * velE * sin(lat);
        e32 = 0;
        e33 =  (((velE^2)/((N+alt)^2)) + ((velN^2)/((M+alt)^2)));
        Fvp = [e11 e12 e13; e21 e22 e23; e31 e32 e33;];
    
        Fpe = zeros(3);
    
        e11 = 1/((M+alt));
        e12 = 0;
        e13 = 0;
        e21 = 0;
        e22 = 1/(((N+alt))*cos(lat));
        e23 = 0;
        e31 = 0;
        e32 = 0;
        e33 = -1;
        Fpv = [e11 e12 e13; e21 e22 e23; e31 e32 e33;];
    
        e11 = 0;
        e12 = 0;
        e13 = -velN/(((M+alt))^2);
        e21 = (velE*tan(lat))/(((N+alt))*cos(lat));
        e22 = 0;
        e23 = -velE/((((N+alt))^2)*cos(lat));
        e31 = 0;
        e32 = 0;
        e33 = 0;
        Fpp = [e11 e12 e13; e21 e22 e23; e31 e32 e33;];
    
    
        %     Fvv = zeros(3);
        %     Fvp = zeros(3);
        %     Fpp = zeros(3);
    
        Fmatrix =  [Fee    Fev    Fep      DCMbn          Z      ;
                    Fve    Fvv    Fvp        Z           DCMbn   ;
                    Fpe    Fpv    Fpp        Z            Z      ;
                    Z      Z      Z          Z            Z      ;
                    Z      Z      Z          Z            Z      ;];


end

== matlab function TRN_V3_2_CodeGen/TRN/ModeManagementCSU_v6/FmatGmatUpdate/Gupdate ==
  data: DCMbn input; Gmatrix output
% ---------------------------------------------------------------------- %
%                   G matrix update function
%
%   INPUT:
%       DCMbn: Rotational matrix(body frame to navigation frame)
%
%   OUTPUT:
%       Gmatrix: Input matrix of Kalman Filter
%
% ---------------------------------------------------------------------- %
function Gmatrix = Gupdate(DCMbn)

Z  = zeros(3);

Gmatrix =  [ -DCMbn     Z;
                Z      DCMbn;
                Z       Z;
                Z       Z;
                Z       Z;];      

end

== matlab function TRN_V3_2_CodeGen/TRN/ModeManagementCSU_v6/TrackingCSUMeasurement/GPSflagcheck ==
  data: FoM input; GPSflag output; EstHorErr input; EstVerErr input; state input; GPSDataNotValid input; AccY input
function GPSflag  = GPScheck(FoM, EstHorErr, EstVerErr, state, GPSDataNotValid, AccY)

GPSflag = uint32(2);

if GPSDataNotValid == 0
%     if EstHorErr < 100 && EstVerErr < 25 && state == 5
        if FoM <= 4
            GPSflag = uint32(1);
            if FoM <= 2 && AccY < 2
                GPSflag = uint32(0);
            end
        end
%    end
else
    GPSflag = uint32(2);
end

== matlab function TRN_V3_2_CodeGen/TRN/ModeManagementCSU_v6/TrackingCSUMeasurement/MesurementUpdate ==
  data: GPSDataNotValid input; Lat_INS input; Lon_INS input; Hmatrix_TRN output; Alt_INS input; RALTAltitude input; z_TRN output; Hmatrix_GPS output; z_GPS output; Lat_GPS input; Lon_GPS input; Alt_GPS input; velN_GPS input; velE_GPS input; velD_GPS input; velN_INS input; velE_INS input; velD_INS input; M input; N input; psi input
function [Hmatrix_TRN, z_TRN, Hmatrix_GPS, z_GPS] = MeasurementUpdate(GPSDataNotValid, Lat_INS, Lon_INS, Alt_INS, RALTAltitude, ...
                                                                      Lat_GPS, Lon_GPS, Alt_GPS, velN_GPS, velE_GPS, velD_GPS, ...
                                                                      velN_INS, velE_INS, velD_INS, ...
                                                                      M, N, psi)

if (GPSDataNotValid == 1)
    P_low = 0.0;
    P_high = 0.0;
    P_left = 0.0;
    P_right = 0.0;
    resultDTED = int32(1);
    resultDVOF = int32(1);
    hDEM = double(0.0);
    Hmatrix_GPS = zeros(6,15);
    z_GPS = zeros(6,1);

    resolution = 3 * 0.000277777777777777;     % DTED Level 1

    Lat_INS = rad2deg(Lat_INS);
    Lon_INS = rad2deg(Lon_INS);

%     resultDVOF = coder.ceval('UpdateObstList', Lat_INS, Lon_INS);
    resultDTED = coder.ceval('UpdateCache', Lat_INS, Lon_INS);

    P_low    =   coder.ceval('MAPGetTerrainHeight', Lat_INS - resolution, Lon_INS);
    P_high   =   coder.ceval('MAPGetTerrainHeight', Lat_INS + resolution, Lon_INS);
    P_left   =   coder.ceval('MAPGetTerrainHeight', Lat_INS             , Lon_INS - resolution);
    P_right  =   coder.ceval('MAPGetTerrainHeight', Lat_INS             , Lon_INS + resolution);

    hdot_lat    =   (P_high - P_low) / resolution;
    hdot_lon    =   (P_right - P_left) / resolution;

    % H matrix
    Hmatrix_TRN =  [ zeros(1,6) -hdot_lat   -hdot_lon    1  zeros(1,6) ];

    hDEM = coder.ceval('MAPGetTerrainHeight', Lat_INS, Lon_INS);

    z_TRN = (Alt_INS - hDEM) - RALTAltitude;

else

    Hmatrix_TRN =  zeros(1,15);
    z_TRN = 0;
    hDEM = double(0.0);
    

    Z   = zeros(3);
    I   = eye(3);
    H   = [(M+Alt_INS)        0             0;
        0     (N+Alt_INS)*cos(psi)     0;
        0            0             1];

    % H matrix
    Hmatrix_GPS = [Z Z H Z Z
                   Z I Z Z Z];


    z_GPS = [(M+Alt_INS)*(Lat_INS-Lat_GPS);
        (N+Alt_INS)*cos(psi)*(Lon_INS-Lon_GPS);
        Alt_INS - Alt_GPS;
        velN_INS - velN_GPS;
        velE_INS - velE_GPS;
        velD_INS - velD_GPS];
end

end

== matlab function TRN_V3_2_CodeGen/TRN/ModeManagementCSU_v6/TrackingCSUMeasurement/MesurementValid ==
  data: GPSDataNotValid input; roll input; pitch input; updateValid input; z_TRN output; zmat_inTRN input; RALTTimeTag input; RALTTimeTag_temp input; RLATvalid input; residualValid input; GPStimeValid input; GPStimeValid_temp input; zmat_inGPS input; GPS_flag input; z_GPS output
function [z_TRN, z_GPS] = MesurementValid(GPSDataNotValid, roll, pitch, updateValid, zmat_inTRN, RALTTimeTag, RALTTimeTag_temp, RLATvalid, ...
                                                        residualValid, GPStimeValid, GPStimeValid_temp, zmat_inGPS, GPS_flag)

z_TRN = 0;
z_GPS = zeros(6,1);

if (GPSDataNotValid == 1)

    z_GPS = zeros(6,1);

    if (updateValid == true && abs(roll) < deg2rad(15) && abs(pitch) < deg2rad(15) && RLATvalid == true && (abs(RALTTimeTag - RALTTimeTag_temp)) > 0.000000001)

        z_TRN = zmat_inTRN;

    else
        z_TRN = 0;
    end

else

    z_TRN = 0;

    if (residualValid == true && abs(roll) < deg2rad(15) && abs(pitch) < deg2rad(15) && (abs(GPStimeValid - GPStimeValid_temp)) > 0.000000001)

        if GPS_flag == 0
            z_GPS = zmat_inGPS;

        elseif GPS_flag == 1

            for i = 1:6
                z_GPS(i) = zmat_inGPS(i);

                if i > 3
                    z_GPS(i) = 0;
                end
            end

        else
            z_GPS = zeros(6,1);
        end

    else
        z_GPS = zeros(6,1);

    end
end

end

== matlab function TRN_V3_2_CodeGen/TRN/ModeManagementCSU_v6/TrackingCSUMeasurement/residualValidCheck2/residualCheck ==
  data: residual input; sigma_3 input; residualValid output; count output; count input
function [residualValid, count] = residualCheck(residual, sigma_3, count)

if abs(residual) > sigma_3
    count = count + 1;
else
    count = 0;
end

if count > 7
    residualValid = boolean(false);
else
    residualValid = boolean(true);
end

== matlab function TRN_V3_2_CodeGen/TRN/ModeManagementCSU_v6/TrackingCSUMeasurement/residualValidCheck2/StdDev ==
  data: x input; std output
function std = StdDev(x)

persistent sumX sumX2 cnt
if (isempty(sumX))
    sumX = 0;
end
if (isempty(sumX2))
    sumX2 = 0;
end
if (isempty(cnt))
    cnt = 0;
end

cnt = cnt + 1;
sumX = sumX + x;
sumX2 = sumX2 + x^2;

var = sumX2/cnt - (sumX/cnt)^2;
std = sqrt(var);
end

== matlab function TRN_V3_2_CodeGen/TRN/ModeManagementCSU_v6/ValidityCheck/ValidityCheck function ==
  data: continuousValid input; TRNEstOfINSLatitudeErr output; TRNEstOfINSLongitudeErr output; TRNEstOfINSAltitudeErr output; AircraftPositionCorrectionValid output; latINSErrTRN input; lonINSErrTRN input; altINSErrTRN input
function [TRNEstOfINSLatitudeErr, TRNEstOfINSLongitudeErr, TRNEstOfINSAltitudeErr, AircraftPositionCorrectionValid] = ValidityCheck(continuousValid, latINSErrTRN, lonINSErrTRN, altINSErrTRN)

if continuousValid == true
    TRNEstOfINSLatitudeErr = latINSErrTRN * 180/pi;
    TRNEstOfINSLongitudeErr = lonINSErrTRN * 180/pi;
    TRNEstOfINSAltitudeErr = altINSErrTRN;
    AircraftPositionCorrectionValid = true;
else
    TRNEstOfINSLatitudeErr = 0.0;
    TRNEstOfINSLongitudeErr = 0.0;
    TRNEstOfINSAltitudeErr = 0.0;
    AircraftPositionCorrectionValid = false;
end
end

== matlab function TRN_V3_2_CodeGen/TRN/Terrain_Func/UpdateCache ==
  data: result output; lat input; lon input; hDEM output
function [result, hDEM] = UpdateCache(lat, lon)
%UpdateCache

% Persistent variables
persistent latPrev lonPrev
if isempty(latPrev)
    latPrev = 0.0;
end
if isempty(lonPrev)
    lonPrev = 0.0;
end

% Initialize output
result = int32(1);
hDEM = double(0.0);

if ( abs(lat - latPrev) > 0.05 ) || ( abs(lon - lonPrev) > 0.05)
    result = coder.ceval('UpdateCache', lat, lon);
    latPrev = lat;
    lonPrev = lon;
else
    
end

hDEM = coder.ceval('MAPGetTerrainHeight', lat, lon);

== matlab function TRN_V3_2_CodeGen/TRN/TRN_visualization /MATLAB Function3 ==
  data: x input; a output; y input
function a = fcn(x,y)

a = sqrt(x^2+y^2);

== matlab function TRN_V3_2_CodeGen/TRN/TRN_visualization /MATLAB Function4 ==
  data: x input; a output; y input
function a = fcn(x,y)

a = sqrt(x^2+y^2);

== matlab function TRN_V3_2_CodeGen/TRN/Terrain_Func/updateFlag ==
  data: AircraftOffTerrainMap input; roughness input; UpdateFlag output
function UpdateFlag = updateFlag(AircraftOffTerrainMap, roughness)

persistent NotupdateCnt
if(isempty(NotupdateCnt))
    NotupdateCnt = 0;
end

if roughness < 1
    NotupdateCnt = NotupdateCnt + 0.04;
else
    NotupdateCnt = 0;
end

if AircraftOffTerrainMap == 1 || NotupdateCnt > 10 * 60   % 10 min
    UpdateFlag = 0;
else
    UpdateFlag = 1;
end

== matlab function TRN_V3_2_CodeGen/TRN/TRN_visualization /Subsystem/UpdateCache ==
  data: result output; lat input; lon input; hDEM output
function [result, hDEM] = UpdateCache(lat, lon)
%UpdateCache

% Persistent variables
persistent latPrev lonPrev
if isempty(latPrev)
    latPrev = 0.0;
end
if isempty(lonPrev)
    lonPrev = 0.0;
end

% Initialize output
result = int32(1);
hDEM = double(0.0);

if ( abs(lat - latPrev) > 0.05 ) || ( abs(lon - lonPrev) > 0.05)
    result = coder.ceval('UpdateCache', lat, lon);
    latPrev = lat;
    lonPrev = lon;
else
    
end

hDEM = coder.ceval('MAPGetTerrainHeight', lat, lon);

== matlab function TRN_V3_2_CodeGen/TRN/TRN_visualization /Subsystem/MATLAB Function ==
  data: Resolution output; Map_Size output; bottomLat output; leftLon output
function [Resolution, Map_Size, bottomLat, leftLon] = ReturnBottomLeftLatLon

Resolution = double(0.0);
Map_Size = double(0.0);

leftLon = 0.0;
leftLon = coder.ceval('ReturnLeftLon');

bottomLat = 0.0;
bottomLat = coder.ceval('ReturnBottomLat');

end
